simulink model "root_param_gimbal"  (R2025b)
settings: Solver=FixedStepAuto  StartTime=0.0  StopTime=10  FixedStep=0.001  RelTol=1e-3
model workspace: external: MATLAB File V1_5GimbalAssembly_DataFile.m (data not in the file)
values from neighbouring files (symbols this model uses):
  X = mk(x(4)*sc,x(5)*sc,x(6)*sc*kdm)    [body_dashboard.m]    (also in run_ga_param.m = mk(g(4),g(5),g(6)); run_gimbal.m = mk(x(4)*sc,  x(5)*sc,  x(6)*sc*kdm))
  Y = mk(x(7)*sc,x(8)*sc,x(9)*sc*kdm)    [body_dashboard.m]    (also in run_ga_param.m = mk(g(7),g(8),g(9)); run_gimbal.m = mk(x(7)*sc,  x(8)*sc,  x(9)*sc*kdm))
  Z = mk(x(10)*sc,x(11)*sc,x(12)*sc)    [body_dashboard.m]    (also in run_ga_param.m = mk(g(10),g(11),g(12)); run_gimbal.m = mk(x(10)*sc, x(11)*sc, x(12)*sc))
undefined symbols (not defined in the file or in its folder): cx, cy, cz, deg, Ixx, Iyy, Izz, Larm, M, rad, s, smiData
libraries: sm_lib x176, nesl_utility x16, eeGeneralControl x3, simulink_extras x2, aerolibconvert2 x1
(part 1 of 4)
settings Model: VariantFading=off  Creator=lew11  LastModifiedBy=rosette-nebula
settings ExplorerConfigSet: InternalSimMechanicsExplorerSettings="<ExplorerConfiguration><canonicalview>default</canonicalview><TilePanel><TileInfo><Tiles Columns=\"1\" Count=\"1\" Height=\"354\" Rows=\"1\" Width=\"500\"><Row Weight=\"1\"/><Column Weight=\"1\"/><Tile Height=\"1\" Width=\"1\" X=\"0\" Y=\"0\"/></Tiles></TileInfo><SceneInfo><SceneViewer><IsThisViewStd><IsStandardView>off</IsStandardView><StandardViewName>Front</StandardViewName></IsThisViewStd><BGColor><R>1</R><G>1</G><B>1</B><A>1</A></BGColor><Camera><DoPerspective>on</DoPerspective><Position><X>58.534417625304727</X><Y>59.860292502851884</Y><Z>-155.4484559381535</Z></Position><Center><X>58.593669358868226</X><Y>61.904700755979775</Y><Z>-155.67104517290912</Z></Center><Up><X>0.0031343571675282087</X><Y>0.10814714230559933</Y><Z>0.99412995700576234</Z></Up><XLim>0.95935498007468478</XLim><YLim>0.95935498007468478</YLim><ViewLimDist>0.01</ViewLimDist></Camera></SceneViewer></SceneInfo></TilePanel><MechEditorPanel><GfxPanelCameraMap><MapElement CameraMLId=\"Camera1\" GfxPanelIndex=\"0\"/></GfxPanelCameraMap><Cameras><Camera><Id>Camera1</Id><Value><Name>Body Cam</Name><NativeCamera><PositionTrackingFeature>Multibody_Sim.Body_Cam.R</PositionTrackingFeature><CenterTrackingFeature>Multibody_Sim.COM_Ref.R</CenterTrackingFeature><UpVectorTrackingFeature>Multibody_Sim.World.W</UpVectorTrackingFeature><CenterTrackingOrigin>on</CenterTrackingOrigin><UpVectorTrackingDirection>+Z</UpVectorTrackingDirection></NativeCamera></Value></Camera><Camera><Id>Camera2</Id><Value><Name>Camera2</Name><NativeCamera><PositionKeyframeSet><Keyframe><Time>0</Time><Value><X>0.11301</X><Y>-1.4589000000000001</Y><Z>0.22284999999999999</Z></Value></Keyframe></PositionKeyframeSet><CenterKeyframeSet><Keyframe><Time>0</Time><Value><X>0.11301</X><Y>-0.55457000000000001</Y><Z>0.22284999999999999</Z></Value></Keyframe></CenterKeyframeSet><UpVectorKeyframeSet><Keyframe><Time>0</Time><Value><X>0</X><Y>0</Y><Z>1</Z></Value></Keyframe></UpVectorKeyframeSet></NativeCamera></Value></Camera><Camera><Id>Camera3</Id><Value><Name>ISO Downwards</Name><NativeCamera><PositionTrackingFeature>Multibody_Sim.TOP.Upper_Structure_Assembly_1_STEP_3_RIGID.F</PositionTrackingFeature><CenterTrackingFeature>Multibody_Sim.Floor_R</CenterTrackingFeature><UpVectorTrackingFeature>Multibody_Sim.Floor_R</UpVectorTrackingFeature><CenterTrackingOrigin>on</CenterTrackingOrigin><UpVectorTrackingDirection>+Z</UpVectorTrackingDirection></NativeCamera></Value></Camera><Camera><Id>Camera4</Id><Value><Name>ISO tracking</Name><NativeCamera><PositionTrackingFeature>Multibody_Sim.World.W</PositionTrackingFeature><CenterTrackingFeature>Multibody_Sim.COM_Ref_R</CenterTrackingFeature><UpVectorTrackingFeature>Multibody_Sim.World_Frame.W</UpVectorTrackingFeature><CenterTrackingOrigin>on</CenterTrackingOrigin><UpVectorTrackingDirection>+Z</UpVectorTrackingDirection></NativeCamera></Value></Camera></Cameras><VideoCreator><IncludeTiles>All</IncludeTiles><IncludeTime>on</IncludeTime><IncludeWorldFrame>off</IncludeWorldFrame><PlaybackSpeedRatio>1</PlaybackSpeedRatio><FrameRate>30</FrameRate><FrameSize>auto</FrameSize><VideoFormat>UncompressedAVI</VideoFormat></VideoCreator></MechEditorPanel><PlaybackSettings><PlaybackSpeedFactor>1</PlaybackSpeedFactor></PlaybackSettings></ExplorerConfiguration>"

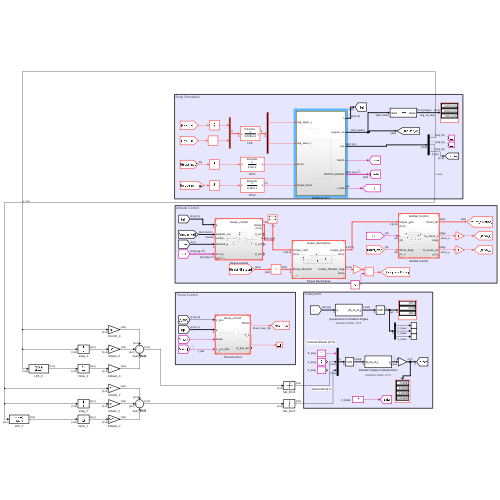
[thumbnail: Simulink's stored preview of the top-level diagram]
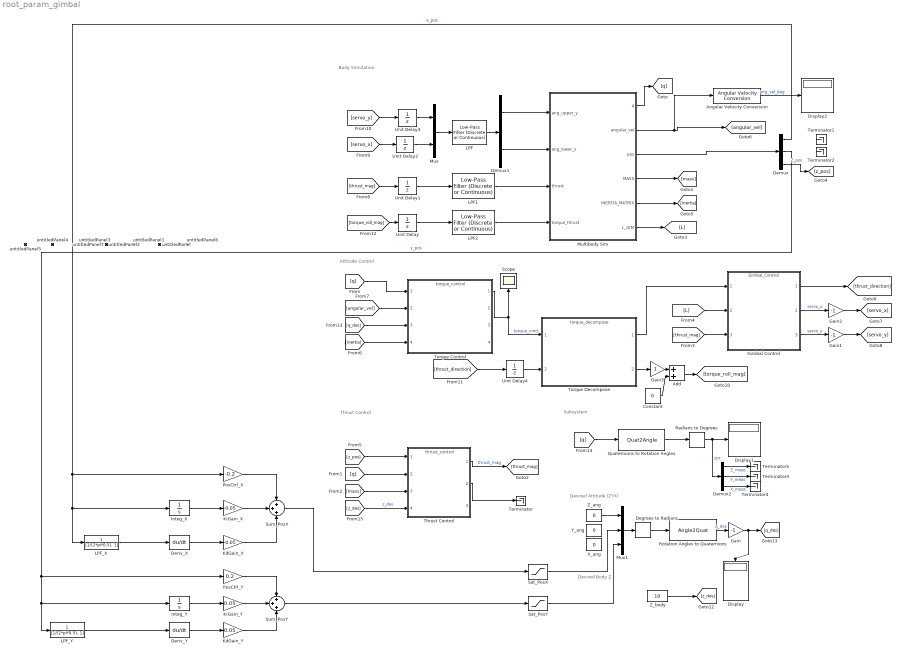
== system root_param_gimbal ==
  note: Subsystem
  note: Body Simulation
  note: Attitude Control
  note: Thrust Control
  note: Desired Body Z
  note: Desired Attitude (ZYX)
  Add : Sum
  Angular Velocity Conversion : aerolibconvert2/Angular Velocity Conversion  IU=rad/s  OU=deg/s
  Constant : Constant  Value=0
  Degrees to Radians : simulink_extras/Transformations/Degrees to Radians
  Demux : Demux  Outputs=3
  Demux1 : Demux  Outputs=2
  Demux2 : Demux  Outputs=3
  Deriv_X : Derivative
  Deriv_Y : Derivative
  Display : Display
  Display1 : Display
  Display2 : Display
  Gain : Gain  Gain=-1
  Gain1 : Gain  Gain=-1
  Gain2 : Gain  Gain=-1
  Gain3 : Gain
  Gimbal Control : ModelReference  ModelNameDialog=Gimbal_Control.slx  SimulationMode=Normal  ModelReferenceVersion=1.54
  Integ_X : Integrator  UpperSaturationLimit=5  LowerSaturationLimit=-5
  Integ_Y : Integrator  UpperSaturationLimit=5  LowerSaturationLimit=-5
  KdGain_X : Gain  Gain=-0.05
  KdGain_Y : Gain  Gain=0.05
  KiGain_X : Gain  Gain=-0.05
  KiGain_Y : Gain  Gain=0.05
  LPF : eeGeneralControl/Low-Pass Filter (Discrete or Continuous)  K=1  T=.016  B=inf  A=-inf  init_option=Inherited from block input  x0=0  Ts=-1
  LPF1 : eeGeneralControl/Low-Pass Filter (Discrete or Continuous)  K=1  T=.3  B=inf  A=-inf  init_option=Inherited from block input  x0=0  Ts=-1
  LPF2 : eeGeneralControl/Low-Pass Filter (Discrete or Continuous)  K=1  T=.15  B=inf  A=-inf  init_option=Inherited from block input  x0=0  Ts=-1
  LPF_X : TransferFcn  Denominator=[1/(2*pi*0.5), 1]
  LPF_Y : TransferFcn  Denominator=[1/(2*pi*0.5), 1]
  Multibody Sim : Subsystem
  Mux : Mux  Inputs=2
  Mux1 : Mux  Inputs=3
  PosCtrl_X : Gain  Gain=-0.2
  PosCtrl_Y : Gain  Gain=0.2
  Quaternions to Rotation Angles : Quat2Angle
      settings: AttributesFormatString=Rotation Order: %<rotationOrder>
  Radians to Degrees : simulink_extras/Transformations/Radians to Degrees
  Rotation Angles to Quaternions : Angle2Quat
      settings: AttributesFormatString=Rotation Order: %<rotationOrder>
  Sat_PosX : Saturate  UpperLimit=5  LowerLimit=-5
  Sat_PosY : Saturate  UpperLimit=5  LowerLimit=-5
  Scope : Scope
      settings: ActiveDisplayYMinimum=-79.161810324182255  ActiveDisplayYMaximum=103.6822961069733
  Sum_PosX : Sum  Inputs=+++
  Sum_PosY : Sum  Inputs=+++
  Terminator{,1..5} (6 alike) : Terminator
  Thrust Control : ModelReference  ModelNameDialog=thrust_control.slx  SimulationMode=Normal  ModelReferenceVersion=3.29
  Torque Control : ModelReference  ModelNameDialog=torque_control  SimulationMode=Normal  ModelReferenceVersion=1.119
  Torque Decompose : ModelReference  ModelNameDialog=torque_decompose.slx  SimulationMode=Normal  ModelReferenceVersion=1.40
  Unit Delay : UnitDelay  SampleTime=-1  HasFrameUpgradeWarning=on
  Unit Delay1 : UnitDelay  InitialCondition=7.559586  SampleTime=-1  HasFrameUpgradeWarning=on
  Unit Delay2 : UnitDelay  SampleTime=-1  HasFrameUpgradeWarning=on
  Unit Delay3 : UnitDelay  SampleTime=-1  HasFrameUpgradeWarning=on
  Unit Delay4 : UnitDelay  InitialCondition=[0; 0; -1]  SampleTime=-1  HasFrameUpgradeWarning=on
  X_ang : Constant  Value=0
  Y_ang : Constant  Value=0
  Z_ang : Constant  Value=0
  Z_body : Constant  Value=10
  untitledPanel : Subsystem  Tag=HiddenForWebPanel  IsWebBlockPanel=on
  untitledPanel1 : Subsystem  Tag=HiddenForWebPanel  IsWebBlockPanel=on
  untitledPanel2 : Subsystem  Tag=HiddenForWebPanel  IsWebBlockPanel=on
  untitledPanel3 : Subsystem  Tag=HiddenForWebPanel  IsWebBlockPanel=on
  untitledPanel4 : Subsystem  Tag=HiddenForWebPanel  IsWebBlockPanel=on
  untitledPanel5 : Subsystem  Tag=HiddenForWebPanel  IsWebBlockPanel=on
  untitledPanel6 : Subsystem  Tag=HiddenForWebPanel  IsWebBlockPanel=on
  untitledPanel7 : Subsystem  Tag=HiddenForWebPanel  IsWebBlockPanel=on
  wires:
  Thrust Control/2 -> Terminator/1
  [z_pos] -> Thrust Control/1
  Thrust Control/1 -> [thrust_mag]  "thrust_mag"
  [mass] -> Thrust Control/3
  [q] -> Thrust Control/2
  [z_des] -> Thrust Control/4  "z_des"
  [q] -> Torque Control/1
  Gimbal Control/3 -> Gain1/1  "servo_y"
  Torque Control/1 -> Scope/1, Torque Decompose/1  "torque_cmd"
  [angular_vel] -> Torque Control/2
  Torque Decompose/1 -> Gimbal Control/1
  Torque Decompose/2 -> Gain3/1
  Gain2/1 -> [servo_x]
  [thrust_direction] -> Unit Delay4/1
  Unit Delay4/1 -> Torque Decompose/2
  [thrust_mag] -> Gimbal Control/3
  Gain1/1 -> [servo_y]
  Gimbal Control/1 -> [thrust_direction]
  [L] -> Gimbal Control/2
  Gimbal Control/2 -> Gain2/1  "servo_x"
  [inertia] -> Torque Control/4
  [q_des] -> Torque Control/3
  Unit Delay1/1 -> LPF1/1
  Demux/3 -> [z_pos]  "Z_pos"
  [servo_x] -> Unit Delay2/1
  LPF1/1 -> Multibody Sim/3(thrust)
  [torque_roll_mag] -> Unit Delay/1
  Unit Delay2/1 -> Mux/2
  Angular Velocity Conversion/1 -> Display2/1  "ang_vel_deg"
  Unit Delay3/1 -> Mux/1
  [thrust_mag] -> Unit Delay1/1
  LPF2/1 -> Multibody Sim/4(torque_thrust)
  Unit Delay/1 -> LPF2/1
  Demux1/1 -> Multibody Sim/1(ang_upper_y)
  Demux1/2 -> Multibody Sim/2(ang_lower_x)
  Mux/1 -> LPF/1
  [servo_y] -> Unit Delay3/1
  LPF/1 -> Demux1/1
  Mux1/1 -> Degrees to Radians/1
  Z_body/1 -> [z_des]
  Demux2/1 -> Terminator5/1  "Z_meas"
  Quaternions to Rotation Angles/1 -> Radians to Degrees/1
  Degrees to Radians/1 -> Rotation Angles to Quaternions/1
  Z_ang/1 -> Mux1/1
  Radians to Degrees/1 -> Demux2/1, Display1/1  "zyx"
  Rotation Angles to Quaternions/1 -> Gain/1  "q_des"
  [q] -> Quaternions to Rotation Angles/1
  Demux2/2 -> Terminator3/1  "Y_meas"
  Demux2/3 -> Terminator4/1  "X_meas"
  Gain3/1 -> Add/1
  Add/1 -> [torque_roll_mag]
  Constant/1 -> Add/2
  Gain/1 -> [q_des], Display/1
  Demux/1 -> Integ_X/1, LPF_X/1, PosCtrl_X/1  "x_pos"
  LPF_X/1 -> Deriv_X/1
  Deriv_X/1 -> KdGain_X/1
  Demux/2 -> PosCtrl_Y/1, Integ_Y/1, LPF_Y/1  "y_pos"
  LPF_Y/1 -> Deriv_Y/1
  Deriv_Y/1 -> KdGain_Y/1
  Integ_X/1 -> KiGain_X/1
  PosCtrl_X/1 -> Sum_PosX/1
  KiGain_X/1 -> Sum_PosX/2
  KdGain_X/1 -> Sum_PosX/3
  Integ_Y/1 -> KiGain_Y/1
  PosCtrl_Y/1 -> Sum_PosY/1
  KiGain_Y/1 -> Sum_PosY/2
  KdGain_Y/1 -> Sum_PosY/3
  Sum_PosX/1 -> Sat_PosX/1
  Sat_PosX/1 -> Mux1/2
  Sum_PosY/1 -> Sat_PosY/1
  Sat_PosY/1 -> Mux1/3
  Multibody Sim/1(q) -> [q]
  Multibody Sim/2(angular_vel) -> Angular Velocity Conversion/1, [angular_vel]
  Multibody Sim/3(pos) -> Demux/1
  Multibody Sim/4(MASS) -> [mass]
  Multibody Sim/5(INERTIA_MATRIX) -> [inertia]
  Multibody Sim/6(L_GIM) -> [L]
